simulink model "SIMULINK_4"  (R2024a)
settings: Solver=VariableStepAuto  StartTime=0.0  StopTime=20  RelTol=1e-3
values from neighbouring files (symbols this model uses):
  L_den = [M B k]    [DAVID_JE_CSE_4.m]
  L_num = [1]    [DAVID_JE_CSE_4.m]
settings Model: Creator=PC  LastModifiedBy=PC

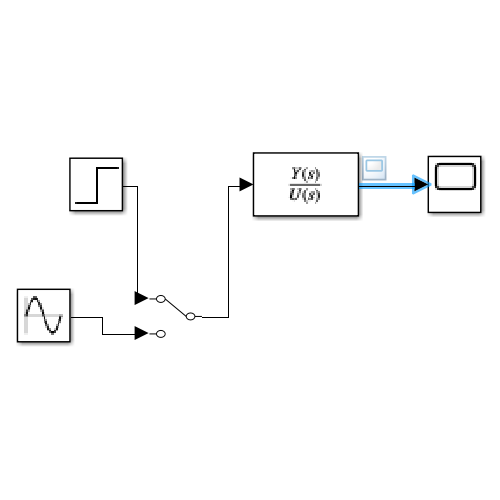
[thumbnail: Simulink's stored preview of the top-level diagram]
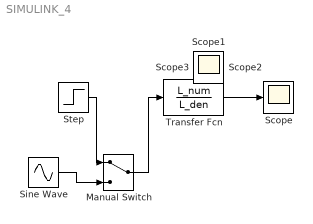
== system SIMULINK_4 ==
  Manual Switch : ManualSwitch
  Scope{,1..3} (4 alike) : Scope
  Sine Wave : Sin  SampleTime=0
  Step : Step  Time=0  Before=0.1  SampleTime=0
  Transfer Fcn : TransferFcn  Numerator=L_num  Denominator=L_den
  wires:
  Step/1 -> Manual Switch/1
  Transfer Fcn/1 -> Scope/1
  Sine Wave/1 -> Manual Switch/2
  Manual Switch/1 -> Transfer Fcn/1
